simulink model "sampleModel15"  (Simulink 9.1)
settings: Solver=VariableStepAuto  StartTime=0.0  StopTime=10.0  RelTol=1e-3
undefined symbols (not defined in the file): DiscIntNeverNeededParam, magnitude, Newton, Raphson
libraries: simulink x26
settings Model: SuppressorTable="22 serialization::archive 11 0 6 0 0 1 8 0 0 0 0 6 0 0 1 0 21 sampleModel15/cfblk25 0 6 0 0 2 8 0 0 0 0 6 41 Simulink:DataType:WarningOverFlowDetected 0 0 0 6 0  0  0 0 0 0 8 20160608 0 0 0 15 23 17 0 1 40 SimulinkFixedPoint:util:Overflowoccurred 0 0 0  0  8 20160608 0 15 23 17 0 1"  Creator=DELL  LastModifiedBy=DELL
settings DataIOCC: SaveFormat=Dataset
settings OptimizationCC: LifeSpan=auto
settings DebuggingCC: UnderspecifiedInitializationDetection=Simplified  MergeDetectMultiDrivingBlocksExec=error  SFUnexpectedBacktrackingDiag=error  SFNoUnconditionalDefaultTransitionDiag=error  SFExecutionAtInitializationDiag=warning
settings HardwareCC: ProdBitPerPointer=64  ProdBitPerSizeT=64  ProdBitPerPtrDiffT=64  ProdLargestAtomicFloat=Float  ProdIntDivRoundTo=Zero  ProdEndianess=LittleEndian  ProdWordSize=64  ProdHWDeviceType=Intel->x86-64 (Windows64)
settings ModelReferenceCC: PropagateSignalLabelsOutOfModel=on
settings CodeAppCC: StateflowObjectComments=off
settings GRTTargetCC: TargetLangStandard=C99 (ISO)  CombineOutputUpdateFcns=on  GRTInterface=off
settings ConfigComp: CovMetricSettings=dwe  CovHtmlReporting=off  CovSaveCumulativeToWorkspaceVar=off  CovSaveSingleToWorkspaceVar=off  CovExternalEMLEnable=on

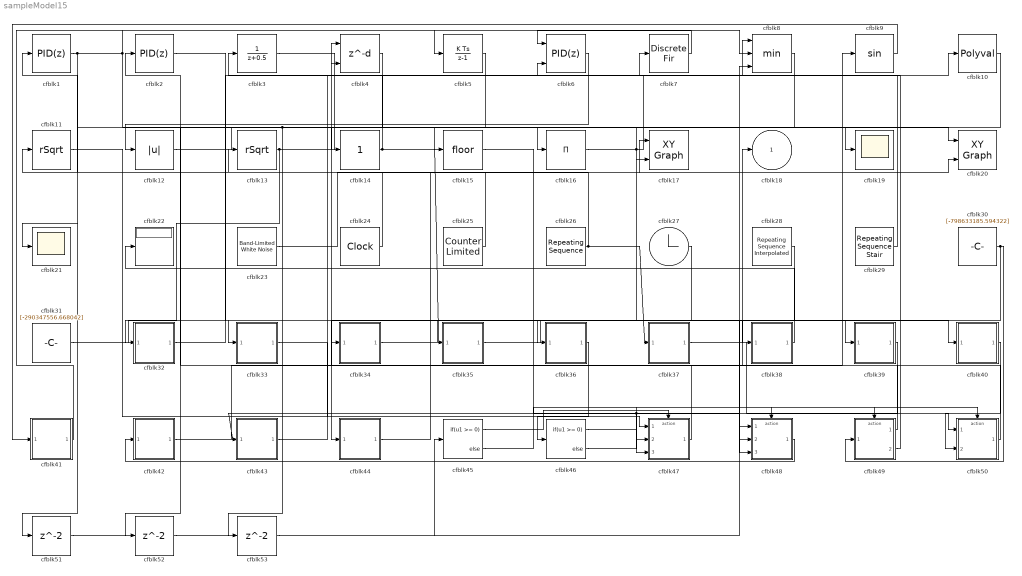
== system sampleModel15 ==
  cfblk1 : simulink/Continuous/PID Controller  Controller=PID  TimeDomain=Discrete-time  SampleTime=1  IntegratorMethod=Forward Euler  FilterMethod=Forward Euler  Form=Parallel  UseFilter=on  ControllerParametersSource=internal  P=1  I=1  D=0  N=100  InitialConditionSource=internal  InitialConditionForIntegrator=0  InitialConditionForFilter=0  ExternalReset=none  LimitOutput=off  UpperSaturationLimit=inf  LowerSaturationLimit=-inf  LinearizeAsGain=off  AntiWindupMode=none  Kb=1  TrackingMode=off  Kt=1  PParamMin=[]  PParamMax=[]  IParamMin=[]  IParamMax=[]  DParamMin=[]  DParamMax=[]  NParamMin=[]  NParamMax=[]  KbParamMin=[]  KbParamMax=[]  KtParamMin=[]  KtParamMax=[]  POutMin=[]  POutMax=[]  IOutMin=[]  IOutMax=[]  DOutMin=[]  DOutMax=[]  NOutMin=[]  NOutMax=[]  KbOutMin=[]  KbOutMax=[]  KtOutMin=[]  KtOutMax=[]  IntegratorOutMin=[]  IntegratorOutMax=[]  FilterOutMin=[]  FilterOutMax=[]  SumOutMin=[]  SumOutMax=[]  SumI1OutMin=[]  SumI1OutMax=[]  SumI2OutMin=[]  SumI2OutMax=[]  SumI3OutMin=[]  SumI3OutMax=[]  SumDOutMin=[]  SumDOutMax=[]  SaturationOutMin=[]  SaturationOutMax=[]  IntegratorContinuousStateAttributes=''  IntegratorStateMustResolveToSignalObject=off  IntegratorRTWStateStorageClass=Auto  FilterContinuousStateAttributes=''  FilterStateMustResolveToSignalObject=off  FilterRTWStateStorageClass=Auto  DifferentiatorICPrevScaledInput=0  DifferentiatorOutMin=[]  DifferentiatorOutMax=[]  FilterDiffOutCoefMin=[]  FilterDiffOutCoefMax=[]  SumDenOutMin=[]  SumDenOutMax=[]  SumNumOutMin=[]  SumNumOutMax=[]  ReciprocalOutMin=[]  ReciprocalOutMax=[]  DivideOutMin=[]  DivideOutMax=[]  TunerSelectOption=Transfer Function Based (PID Tuner App)
  cfblk10 : Polyval  Coefs=[ +2.081618890e-019, -1.441693666e-014, +4.719686976e-010, -8.536869453e-006, +1.621573104e-001, -8.087801117e+001 ]
  cfblk11 : Sqrt  Operator=rSqrt  AlgorithmType=Newton-Raphson  SaturateOnIntegerOverflow=on
  cfblk12 : Abs
  cfblk13 : Sqrt  Operator=rSqrt  AlgorithmType=Newton-Raphson  SaturateOnIntegerOverflow=on
  cfblk14 : simulink/Math Operations/Slider Gain  gain=1  low=0  high=2
  cfblk15 : Rounding
  cfblk16 : Product  Inputs=*
  cfblk17 : simulink/Sinks/XY Graph  xmin=-1  xmax=1  ymin=-1  ymax=1  st=-1
  cfblk19 : Scope
  cfblk2 : simulink/Continuous/PID Controller  Controller=PID  TimeDomain=Discrete-time  SampleTime=1  IntegratorMethod=Forward Euler  FilterMethod=Forward Euler  Form=Parallel  UseFilter=on  ControllerParametersSource=internal  P=1  I=1  D=0  N=100  InitialConditionSource=internal  InitialConditionForIntegrator=0  InitialConditionForFilter=0  ExternalReset=none  LimitOutput=off  UpperSaturationLimit=inf  LowerSaturationLimit=-inf  LinearizeAsGain=off  AntiWindupMode=none  Kb=1  TrackingMode=off  Kt=1  PParamMin=[]  PParamMax=[]  IParamMin=[]  IParamMax=[]  DParamMin=[]  DParamMax=[]  NParamMin=[]  NParamMax=[]  KbParamMin=[]  KbParamMax=[]  KtParamMin=[]  KtParamMax=[]  POutMin=[]  POutMax=[]  IOutMin=[]  IOutMax=[]  DOutMin=[]  DOutMax=[]  NOutMin=[]  NOutMax=[]  KbOutMin=[]  KbOutMax=[]  KtOutMin=[]  KtOutMax=[]  IntegratorOutMin=[]  IntegratorOutMax=[]  FilterOutMin=[]  FilterOutMax=[]  SumOutMin=[]  SumOutMax=[]  SumI1OutMin=[]  SumI1OutMax=[]  SumI2OutMin=[]  SumI2OutMax=[]  SumI3OutMin=[]  SumI3OutMax=[]  SumDOutMin=[]  SumDOutMax=[]  SaturationOutMin=[]  SaturationOutMax=[]  IntegratorContinuousStateAttributes=''  IntegratorStateMustResolveToSignalObject=off  IntegratorRTWStateStorageClass=Auto  FilterContinuousStateAttributes=''  FilterStateMustResolveToSignalObject=off  FilterRTWStateStorageClass=Auto  DifferentiatorICPrevScaledInput=0  DifferentiatorOutMin=[]  DifferentiatorOutMax=[]  FilterDiffOutCoefMin=[]  FilterDiffOutCoefMax=[]  SumDenOutMin=[]  SumDenOutMax=[]  SumNumOutMin=[]  SumNumOutMax=[]  ReciprocalOutMin=[]  ReciprocalOutMax=[]  DivideOutMin=[]  DivideOutMax=[]  TunerSelectOption=Transfer Function Based (PID Tuner App)
  cfblk20 : simulink/Sinks/XY Graph  xmin=-1  xmax=1  ymin=-1  ymax=1  st=-1
  cfblk21 : Scope
  cfblk22 : Display
  cfblk23 : simulink/Sources/Band-Limited White Noise  Cov=[4615233474.301985]  Ts=0.1  seed=[9049221695.000000]
  cfblk24 : DigitalClock
  cfblk25 : simulink/Sources/Counter Limited  uplimit=[387.000000]  tsamp=-1
  cfblk26 : simulink/Sources/Repeating Sequence  rep_seq_t=[0 2]  rep_seq_y=[206033104.560979, 120638017.420712]
  cfblk27 : Clock
  cfblk28 : simulink/Sources/Repeating Sequence Interpolated  OutValues=[691679511.220975, -430390090.474105, 326636995.361738, 204516353.053731, 312925893.425582]  TimeValues=[0 0.1 0.5 0.6 1].'  LookUpMeth=Use Input Nearest  tsamp=0.01  OutMin=[]  OutMax=[]  OutDataTypeStr=double  OutputDataTypeScalingMode=double  OutDataType=fixdt(0,8)  OutScaling=2^-10
  cfblk29 : simulink/Sources/Repeating Sequence Stair  OutValues=[-336712385.924395, -623605342.299720]  tsamp=-1  OutMin=[]  OutMax=[]  OutDataTypeStr=double  OutputDataTypeScalingMode=double  OutDataType=fixdt(0,8)  ConRadixGroup=Best Precision: Vector-wise  OutScaling=2^-12
  cfblk3 : DiscreteTransferFcn  SampleTime=1
  cfblk30 : Constant  Value=[-798633185.594322]  SampleTime=1
  cfblk31 : Constant  Value=[-290347556.668042]  SampleTime=1
  cfblk32 : Subsystem
  cfblk33 : Subsystem
  cfblk34 : Subsystem
  cfblk35 : Subsystem
  cfblk36 : Subsystem
  cfblk37 : Subsystem
  cfblk38 : Subsystem
  cfblk39 : Subsystem
  cfblk4 : Delay  DelayLengthSource=Input port  SampleTime=1
      settings: InputPortMap=u0,p1
  cfblk40 : Subsystem
  cfblk41 : Subsystem
  cfblk42 : Subsystem
  cfblk43 : Subsystem
  cfblk44 : Subsystem
  cfblk45 : If  IfExpression=u1 >= 0  SampleTime=1
  cfblk46 : If  IfExpression=u1 >= 0  SampleTime=1
  cfblk47 : Subsystem  TreatAsAtomicUnit=on
  cfblk48 : Subsystem  TreatAsAtomicUnit=on
  cfblk49 : Subsystem  TreatAsAtomicUnit=on
  cfblk5 : DiscreteIntegrator  ICPrevOutput=DiscIntNeverNeededParam  ICPrevScaledInput=DiscIntNeverNeededParam
  cfblk50 : Subsystem  TreatAsAtomicUnit=on
  cfblk51 : Delay  SampleTime=1
  cfblk52 : Delay  SampleTime=1
  cfblk53 : Delay  SampleTime=1
  cfblk6 : simulink/Continuous/PID Controller (2DOF)  Controller=PID  TimeDomain=Discrete-time  SampleTime=1  IntegratorMethod=Forward Euler  FilterMethod=Forward Euler  Form=Parallel  UseFilter=on  ControllerParametersSource=internal  P=1  I=1  D=0  N=100  b=1  c=1  InitialConditionSource=internal  InitialConditionForIntegrator=0  InitialConditionForFilter=0  ExternalReset=none  LimitOutput=off  UpperSaturationLimit=inf  LowerSaturationLimit=-inf  LinearizeAsGain=off  AntiWindupMode=none  Kb=1  TrackingMode=off  Kt=1  PParamMin=[]  PParamMax=[]  IParamMin=[]  IParamMax=[]  DParamMin=[]  DParamMax=[]  NParamMin=[]  NParamMax=[]  bParamMin=[]  bParamMax=[]  cParamMin=[]  cParamMax=[]  KbParamMin=[]  KbParamMax=[]  KtParamMin=[]  KtParamMax=[]  POutMin=[]  POutMax=[]  IOutMin=[]  IOutMax=[]  DOutMin=[]  DOutMax=[]  NOutMin=[]  NOutMax=[]  bOutMin=[]  bOutMax=[]  cOutMin=[]  cOutMax=[]  KbOutMin=[]  KbOutMax=[]  KtOutMin=[]  KtOutMax=[]  IntegratorOutMin=[]  IntegratorOutMax=[]  FilterOutMin=[]  FilterOutMax=[]  SumOutMin=[]  SumOutMax=[]  Sum1OutMin=[]  Sum1OutMax=[]  Sum2OutMin=[]  Sum2OutMax=[]  Sum3OutMin=[]  Sum3OutMax=[]  SumI1OutMin=[]  SumI1OutMax=[]  SumI2OutMin=[]  SumI2OutMax=[]  SumI3OutMin=[]  SumI3OutMax=[]  SumDOutMin=[]  SumDOutMax=[]  SaturationOutMin=[]  SaturationOutMax=[]  IntegratorContinuousStateAttributes=''  IntegratorStateMustResolveToSignalObject=off  IntegratorRTWStateStorageClass=Auto  FilterContinuousStateAttributes=''  FilterStateMustResolveToSignalObject=off  FilterRTWStateStorageClass=Auto  DifferentiatorICPrevScaledInput=0  DifferentiatorOutMin=[]  DifferentiatorOutMax=[]  FilterDiffOutCoefMin=[]  FilterDiffOutCoefMax=[]  SumDenOutMin=[]  SumDenOutMax=[]  SumNumOutMin=[]  SumNumOutMax=[]  ReciprocalOutMin=[]  ReciprocalOutMax=[]  DivideOutMin=[]  DivideOutMax=[]  TunerSelectOption=Transfer Function Based (PID Tuner App)
  cfblk7 : DiscreteFir  SampleTime=1
  cfblk8 : MinMax  Inputs=3
  cfblk9 : Trigonometry
  cfblk18 : Outport
  wires:
  cfblk25/1 -> cfblk11/1
  cfblk48/1(cfblk2) -> cfblk42/1(cfblk1)
  cfblk13/1 -> cfblk20/1, cfblk32/1(cfblk1)
  cfblk12/1 -> cfblk19/1
  cfblk6/1 -> cfblk12/1
  cfblk29/1 -> cfblk7/1
  cfblk47/1(cfblk2) -> cfblk4/1
  cfblk7/1 -> cfblk6/1
  cfblk35/1(cfblk2) -> cfblk39/1(cfblk1)
  cfblk3/1 -> cfblk16/1
  cfblk24/1 -> cfblk1/1
  cfblk27/1 -> cfblk44/1(cfblk1)
  cfblk41/1(cfblk2) -> cfblk5/1
  cfblk26/1 -> cfblk37/1(cfblk1), cfblk13/1
  cfblk31/1 -> cfblk33/1(cfblk1)
  cfblk34/1(cfblk2) -> cfblk36/1(cfblk1)
  cfblk42/1(cfblk2) -> cfblk9/1
  cfblk16/1 -> cfblk10/1, cfblk40/1(cfblk1)
  cfblk10/1 -> cfblk14/1
  cfblk49/1(cfblk2) -> cfblk2/1
  cfblk28/1 -> cfblk34/1(cfblk1)
  cfblk14/1 -> cfblk35/1(cfblk1), cfblk4/2
  cfblk50/1(cfblk2) -> cfblk18/1
  cfblk38/1(cfblk2) -> cfblk22/1
  cfblk39/1(cfblk2) -> cfblk43/1(cfblk1), cfblk47/3(cfblk11)
  cfblk8/1 -> cfblk15/1
  cfblk5/1 -> cfblk52/1, cfblk53/1
  cfblk37/1(cfblk2) -> cfblk50/1(cfblk1)
  cfblk43/1(cfblk2) -> cfblk6/2
  cfblk30/1 -> cfblk49/1(cfblk1), cfblk48/3(cfblk7)
  cfblk23/1 -> cfblk20/2
  cfblk9/1 -> cfblk41/1(cfblk1)
  cfblk49/2(cfblk15) -> cfblk3/1
  cfblk40/1(cfblk2) -> cfblk50/2(cfblk12)
  cfblk15/1 -> cfblk48/2(cfblk6)
  cfblk32/1(cfblk2) -> cfblk8/1
  cfblk36/1(cfblk2) -> cfblk46/1
  cfblk33/1(cfblk2) -> cfblk47/1(cfblk1)
  cfblk2/1 -> cfblk38/1(cfblk1)
  cfblk44/1(cfblk2) -> cfblk17/1
  cfblk1/1 -> cfblk17/2, cfblk8/2, cfblk21/1
  cfblk11/1 -> cfblk47/2(cfblk10)
  cfblk45/1 -> cfblk47/Action
  cfblk45/2 -> cfblk48/Action
  cfblk46/1 -> cfblk49/Action
  cfblk46/2 -> cfblk50/Action
  cfblk4/1 -> cfblk51/1
  cfblk51/1 -> cfblk48/1(cfblk1)
  cfblk52/1 -> cfblk45/1
  cfblk53/1 -> cfblk8/3

== system sampleModel15/cfblk32 ==
  cfblk1 : Inport
  cfblk2 : Outport
  wires:
  cfblk1/1 -> cfblk2/1

== system sampleModel15/cfblk33 ==
  cfblk1 : Inport
  cfblk2 : Outport
  wires:
  cfblk1/1 -> cfblk2/1

== system sampleModel15/cfblk34 ==
  cfblk1 : Inport
  cfblk2 : Outport
  wires:
  cfblk1/1 -> cfblk2/1

== system sampleModel15/cfblk35 ==
  cfblk1 : Inport
  cfblk2 : Outport
  wires:
  cfblk1/1 -> cfblk2/1

== system sampleModel15/cfblk36 ==
  cfblk1 : Inport
  cfblk2 : Outport
  wires:
  cfblk1/1 -> cfblk2/1

== system sampleModel15/cfblk37 ==
  cfblk1 : Inport
  cfblk2 : Outport
  wires:
  cfblk1/1 -> cfblk2/1

== system sampleModel15/cfblk38 ==
  cfblk1 : Inport
  cfblk2 : Outport
  wires:
  cfblk1/1 -> cfblk2/1

== system sampleModel15/cfblk39 ==
  cfblk1 : Inport
  cfblk2 : Outport
  wires:
  cfblk1/1 -> cfblk2/1

== system sampleModel15/cfblk40 ==
  cfblk1 : Inport
  cfblk2 : Outport
  wires:
  cfblk1/1 -> cfblk2/1

== system sampleModel15/cfblk41 ==
  cfblk1 : Inport
  cfblk2 : Outport
  wires:
  cfblk1/1 -> cfblk2/1

== system sampleModel15/cfblk42 ==
  cfblk1 : Inport
  cfblk2 : Outport
  wires:
  cfblk1/1 -> cfblk2/1

== system sampleModel15/cfblk43 ==
  cfblk1 : Inport
  cfblk2 : Outport
  wires:
  cfblk1/1 -> cfblk2/1

== system sampleModel15/cfblk44 ==
  cfblk1 : Inport
  cfblk2 : Outport
  wires:
  cfblk1/1 -> cfblk2/1

== system sampleModel15/cfblk47 ==
  cfblk1 : Inport
  cfblk10 : Inport  Port=2
  cfblk11 : Inport  Port=3
  Action Port : ActionPort  ActionType=then
  cfblk12 : Delay
  cfblk3 : Delay
  cfblk4 : DiscreteZeroPole  Poles=[0 0.5]  Gain=1  SampleTime=-1
  cfblk5 : simulink/Continuous/PID Controller  Controller=PID  TimeDomain=Discrete-time  SampleTime=-1  IntegratorMethod=Forward Euler  FilterMethod=Forward Euler  Form=Parallel  UseFilter=on  ControllerParametersSource=internal  P=1  I=1  D=0  N=100  InitialConditionSource=internal  InitialConditionForIntegrator=0  InitialConditionForFilter=0  ExternalReset=none  LimitOutput=off  UpperSaturationLimit=inf  LowerSaturationLimit=-inf  LinearizeAsGain=off  AntiWindupMode=none  Kb=1  TrackingMode=off  Kt=1  PParamMin=[]  PParamMax=[]  IParamMin=[]  IParamMax=[]  DParamMin=[]  DParamMax=[]  NParamMin=[]  NParamMax=[]  KbParamMin=[]  KbParamMax=[]  KtParamMin=[]  KtParamMax=[]  POutMin=[]  POutMax=[]  IOutMin=[]  IOutMax=[]  DOutMin=[]  DOutMax=[]  NOutMin=[]  NOutMax=[]  KbOutMin=[]  KbOutMax=[]  KtOutMin=[]  KtOutMax=[]  IntegratorOutMin=[]  IntegratorOutMax=[]  FilterOutMin=[]  FilterOutMax=[]  SumOutMin=[]  SumOutMax=[]  SumI1OutMin=[]  SumI1OutMax=[]  SumI2OutMin=[]  SumI2OutMax=[]  SumI3OutMin=[]  SumI3OutMax=[]  SumDOutMin=[]  SumDOutMax=[]  SaturationOutMin=[]  SaturationOutMax=[]  IntegratorContinuousStateAttributes=''  IntegratorStateMustResolveToSignalObject=off  IntegratorRTWStateStorageClass=Auto  FilterContinuousStateAttributes=''  FilterStateMustResolveToSignalObject=off  FilterRTWStateStorageClass=Auto  DifferentiatorICPrevScaledInput=0  DifferentiatorOutMin=[]  DifferentiatorOutMax=[]  FilterDiffOutCoefMin=[]  FilterDiffOutCoefMax=[]  SumDenOutMin=[]  SumDenOutMax=[]  SumNumOutMin=[]  SumNumOutMax=[]  ReciprocalOutMin=[]  ReciprocalOutMax=[]  DivideOutMin=[]  DivideOutMax=[]  TunerSelectOption=Transfer Function Based (PID Tuner App)
  cfblk6 : ComplexToMagnitudeAngle
  cfblk7 : Constant  Value=[-442457058.559597]  SampleTime=1
  cfblk8 : Constant  Value=[-425591701.658393]  SampleTime=1
  cfblk9 : Subsystem
  cfblk2 : Outport
  wires:
  cfblk5/1 -> cfblk9/1(cfblk1)
  cfblk4/1 -> cfblk5/1
  cfblk9/1(cfblk2) -> cfblk6/1
  cfblk1/1 -> cfblk2/1
  cfblk6/2 -> cfblk3/1
  cfblk6/1 -> cfblk12/1
  cfblk12/1 -> cfblk4/1

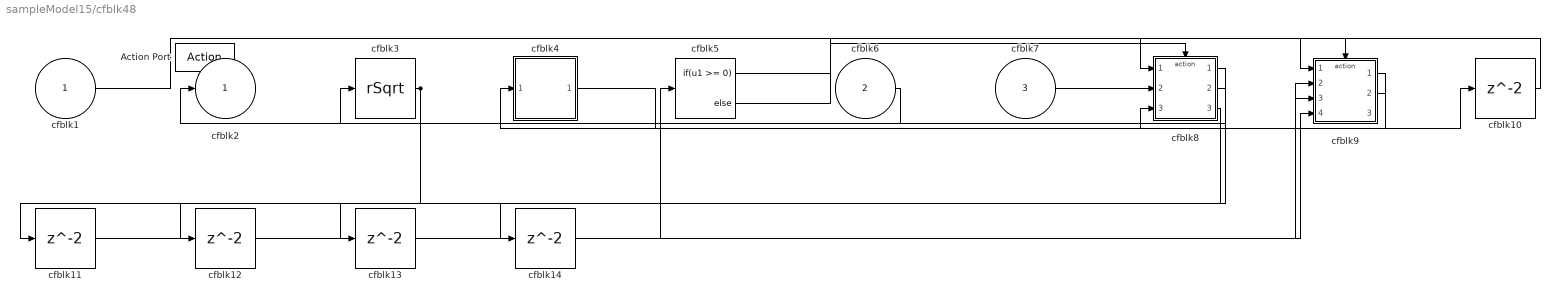
== system sampleModel15/cfblk48 ==
  cfblk1 : Inport
  cfblk6 : Inport  Port=2
  cfblk7 : Inport  Port=3
  Action Port : ActionPort  ActionType=else
  cfblk{10..14} (5 alike) : Delay
  cfblk3 : Sqrt  Operator=rSqrt  AlgorithmType=Newton-Raphson  SaturateOnIntegerOverflow=on
  cfblk4 : Subsystem
  cfblk5 : If  IfExpression=u1 >= 0  SampleTime=1
  cfblk8 : Subsystem  TreatAsAtomicUnit=on
  cfblk9 : Subsystem  TreatAsAtomicUnit=on
  cfblk2 : Outport
  wires:
  cfblk7/1 -> cfblk8/2(cfblk12)
  cfblk1/1 -> cfblk9/1(cfblk1)
  cfblk3/1 -> cfblk12/1, cfblk13/1
  cfblk9/1(cfblk2) -> cfblk4/1(cfblk1)
  cfblk6/1 -> cfblk2/1
  cfblk9/2(cfblk15) -> cfblk8/3(cfblk13)
  cfblk8/2(cfblk14) -> cfblk3/1
  cfblk5/1 -> cfblk8/Action
  cfblk5/2 -> cfblk9/Action
  cfblk4/1(cfblk2) -> cfblk10/1
  cfblk10/1 -> cfblk8/1(cfblk1)
  cfblk8/1(cfblk2) -> cfblk11/1
  cfblk11/1 -> cfblk9/2(cfblk12)
  cfblk12/1 -> cfblk5/1
  cfblk13/1 -> cfblk9/4(cfblk14)
  cfblk8/3(cfblk15) -> cfblk14/1
  cfblk14/1 -> cfblk9/3(cfblk13)

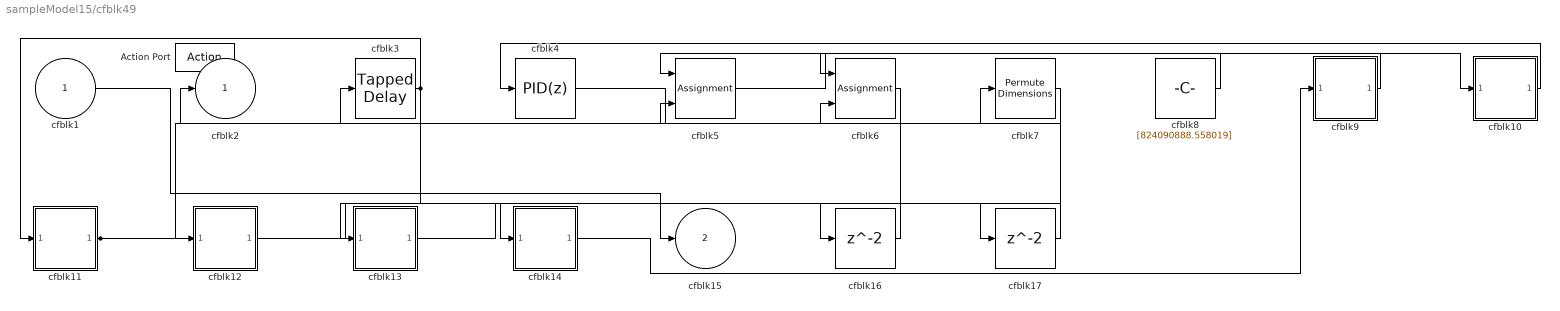
== system sampleModel15/cfblk49 ==
  cfblk1 : Inport
  Action Port : ActionPort  ActionType=then
  cfblk10 : Subsystem
  cfblk11 : Subsystem
  cfblk12 : Subsystem
  cfblk13 : Subsystem
  cfblk14 : Subsystem
  cfblk16 : Delay
  cfblk17 : Delay
  cfblk3 : simulink/Discrete/Tapped Delay  vinit=0.0  samptime=-1  NumDelays=1  DelayOrder=Oldest  includeCurrent=off
  cfblk4 : simulink/Continuous/PID Controller  Controller=PID  TimeDomain=Discrete-time  SampleTime=-1  IntegratorMethod=Forward Euler  FilterMethod=Forward Euler  Form=Parallel  UseFilter=on  ControllerParametersSource=internal  P=1  I=1  D=0  N=100  InitialConditionSource=internal  InitialConditionForIntegrator=0  InitialConditionForFilter=0  ExternalReset=none  LimitOutput=off  UpperSaturationLimit=inf  LowerSaturationLimit=-inf  LinearizeAsGain=off  AntiWindupMode=none  Kb=1  TrackingMode=off  Kt=1  PParamMin=[]  PParamMax=[]  IParamMin=[]  IParamMax=[]  DParamMin=[]  DParamMax=[]  NParamMin=[]  NParamMax=[]  KbParamMin=[]  KbParamMax=[]  KtParamMin=[]  KtParamMax=[]  POutMin=[]  POutMax=[]  IOutMin=[]  IOutMax=[]  DOutMin=[]  DOutMax=[]  NOutMin=[]  NOutMax=[]  KbOutMin=[]  KbOutMax=[]  KtOutMin=[]  KtOutMax=[]  IntegratorOutMin=[]  IntegratorOutMax=[]  FilterOutMin=[]  FilterOutMax=[]  SumOutMin=[]  SumOutMax=[]  SumI1OutMin=[]  SumI1OutMax=[]  SumI2OutMin=[]  SumI2OutMax=[]  SumI3OutMin=[]  SumI3OutMax=[]  SumDOutMin=[]  SumDOutMax=[]  SaturationOutMin=[]  SaturationOutMax=[]  IntegratorContinuousStateAttributes=''  IntegratorStateMustResolveToSignalObject=off  IntegratorRTWStateStorageClass=Auto  FilterContinuousStateAttributes=''  FilterStateMustResolveToSignalObject=off  FilterRTWStateStorageClass=Auto  DifferentiatorICPrevScaledInput=0  DifferentiatorOutMin=[]  DifferentiatorOutMax=[]  FilterDiffOutCoefMin=[]  FilterDiffOutCoefMax=[]  SumDenOutMin=[]  SumDenOutMax=[]  SumNumOutMin=[]  SumNumOutMax=[]  ReciprocalOutMin=[]  ReciprocalOutMax=[]  DivideOutMin=[]  DivideOutMax=[]  TunerSelectOption=Transfer Function Based (PID Tuner App)
  cfblk5 : Assignment  DiagnosticForDimensions=Warning  IndexOptions=Index vector (dialog)  Indices=1  OutputSizes=1
  cfblk6 : Assignment  DiagnosticForDimensions=Warning  IndexOptions=Index vector (dialog)  Indices=1  OutputSizes=1
  cfblk7 : PermuteDimensions
  cfblk8 : Constant  Value=[824090888.558019]  SampleTime=1
  cfblk9 : Subsystem
  cfblk2 : Outport
  cfblk15 : Outport  Port=2
  wires:
  cfblk11/1(cfblk2) -> cfblk12/1(cfblk1), cfblk6/2
  cfblk6/1 -> cfblk2/1
  cfblk3/1 -> cfblk11/1(cfblk1), cfblk13/1(cfblk1)
  cfblk5/1 -> cfblk10/1(cfblk1)
  cfblk12/1(cfblk2) -> cfblk14/1(cfblk1)
  cfblk8/1 -> cfblk6/1
  cfblk1/1 -> cfblk15/1
  cfblk9/1(cfblk2) -> cfblk5/1
  cfblk4/1 -> cfblk7/1
  cfblk10/1(cfblk2) -> cfblk4/1
  cfblk14/1(cfblk2) -> cfblk9/1(cfblk1)
  cfblk7/1 -> cfblk16/1
  cfblk16/1 -> cfblk5/2
  cfblk13/1(cfblk2) -> cfblk17/1
  cfblk17/1 -> cfblk3/1

== system sampleModel15/cfblk50 ==
  cfblk1 : Inport
  cfblk12 : Inport  Port=2
  Action Port : ActionPort  ActionType=else
  cfblk10 : Subsystem
  cfblk11 : Subsystem
  cfblk13 : Delay
  cfblk3 : UnitDelay  SampleTime=-1
  cfblk4 : Sum  Inputs=-+
  cfblk5 : ComplexToMagnitudeAngle
  cfblk6 : simulink/Math Operations/MinMax Running Resettable  Function=min  vinit=0.0
  cfblk7 : Assignment  DiagnosticForDimensions=Warning  IndexOptions=Index vector (dialog)  Indices=1  OutputSizes=1
  cfblk8 : Constant  Value=[310628600.138073]  SampleTime=1
  cfblk9 : Constant  Value=[-993756271.282597]  SampleTime=1
  cfblk2 : Outport
  wires:
  cfblk10/1(cfblk2) -> cfblk2/1
  cfblk11/1(cfblk2) -> cfblk4/1
  cfblk6/1 -> cfblk7/1
  cfblk1/1 -> cfblk5/1
  cfblk8/1 -> cfblk11/1(cfblk1)
  cfblk3/1 -> cfblk4/2
  cfblk12/1 -> cfblk3/1
  cfblk5/1 -> cfblk6/1
  cfblk4/1 -> cfblk10/1(cfblk1)
  cfblk9/1 -> cfblk7/2
  cfblk7/1 -> cfblk13/1
  cfblk13/1 -> cfblk6/2

== system sampleModel15/cfblk47/cfblk9 ==
  cfblk1 : Inport
  cfblk2 : Outport
  wires:
  cfblk1/1 -> cfblk2/1

== system sampleModel15/cfblk48/cfblk4 ==
  cfblk1 : Inport
  cfblk2 : Outport
  wires:
  cfblk1/1 -> cfblk2/1

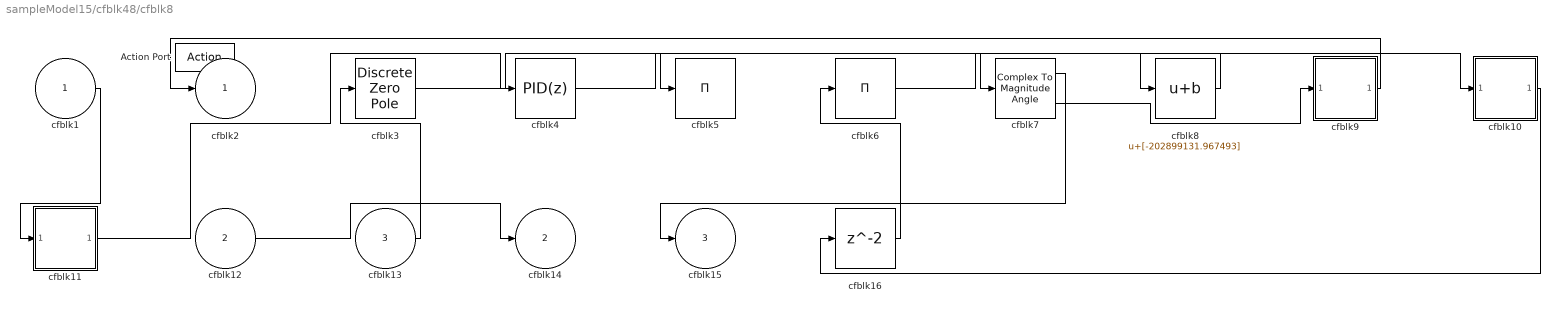
== system sampleModel15/cfblk48/cfblk8 ==
  cfblk1 : Inport
  cfblk12 : Inport  Port=2
  cfblk13 : Inport  Port=3
  Action Port : ActionPort  ActionType=then
  cfblk10 : Subsystem
  cfblk11 : Subsystem
  cfblk16 : Delay
  cfblk3 : DiscreteZeroPole  Poles=[0 0.5]  Gain=1  SampleTime=-1
  cfblk4 : simulink/Continuous/PID Controller  Controller=PID  TimeDomain=Discrete-time  SampleTime=-1  IntegratorMethod=Forward Euler  FilterMethod=Forward Euler  Form=Parallel  UseFilter=on  ControllerParametersSource=internal  P=1  I=1  D=0  N=100  InitialConditionSource=internal  InitialConditionForIntegrator=0  InitialConditionForFilter=0  ExternalReset=none  LimitOutput=off  UpperSaturationLimit=inf  LowerSaturationLimit=-inf  LinearizeAsGain=off  AntiWindupMode=none  Kb=1  TrackingMode=off  Kt=1  PParamMin=[]  PParamMax=[]  IParamMin=[]  IParamMax=[]  DParamMin=[]  DParamMax=[]  NParamMin=[]  NParamMax=[]  KbParamMin=[]  KbParamMax=[]  KtParamMin=[]  KtParamMax=[]  POutMin=[]  POutMax=[]  IOutMin=[]  IOutMax=[]  DOutMin=[]  DOutMax=[]  NOutMin=[]  NOutMax=[]  KbOutMin=[]  KbOutMax=[]  KtOutMin=[]  KtOutMax=[]  IntegratorOutMin=[]  IntegratorOutMax=[]  FilterOutMin=[]  FilterOutMax=[]  SumOutMin=[]  SumOutMax=[]  SumI1OutMin=[]  SumI1OutMax=[]  SumI2OutMin=[]  SumI2OutMax=[]  SumI3OutMin=[]  SumI3OutMax=[]  SumDOutMin=[]  SumDOutMax=[]  SaturationOutMin=[]  SaturationOutMax=[]  IntegratorContinuousStateAttributes=''  IntegratorStateMustResolveToSignalObject=off  IntegratorRTWStateStorageClass=Auto  FilterContinuousStateAttributes=''  FilterStateMustResolveToSignalObject=off  FilterRTWStateStorageClass=Auto  DifferentiatorICPrevScaledInput=0  DifferentiatorOutMin=[]  DifferentiatorOutMax=[]  FilterDiffOutCoefMin=[]  FilterDiffOutCoefMax=[]  SumDenOutMin=[]  SumDenOutMax=[]  SumNumOutMin=[]  SumNumOutMax=[]  ReciprocalOutMin=[]  ReciprocalOutMax=[]  DivideOutMin=[]  DivideOutMax=[]  TunerSelectOption=Transfer Function Based (PID Tuner App)
  cfblk5 : Product  Inputs=*
  cfblk6 : Product  Inputs=*
  cfblk7 : ComplexToMagnitudeAngle
  cfblk8 : Bias  Bias=[-202899131.967493]
  cfblk9 : Subsystem
  cfblk2 : Outport
  cfblk14 : Outport  Port=2
  cfblk15 : Outport  Port=3
  wires:
  cfblk12/1 -> cfblk14/1
  cfblk8/1 -> cfblk7/1
  cfblk7/1 -> cfblk15/1
  cfblk7/2 -> cfblk9/1(cfblk1)
  cfblk3/1 -> cfblk5/1
  cfblk4/1 -> cfblk8/1
  cfblk13/1 -> cfblk3/1
  cfblk9/1(cfblk2) -> cfblk2/1
  cfblk1/1 -> cfblk11/1(cfblk1)
  cfblk11/1(cfblk2) -> cfblk4/1
  cfblk6/1 -> cfblk10/1(cfblk1)
  cfblk10/1(cfblk2) -> cfblk16/1
  cfblk16/1 -> cfblk6/1

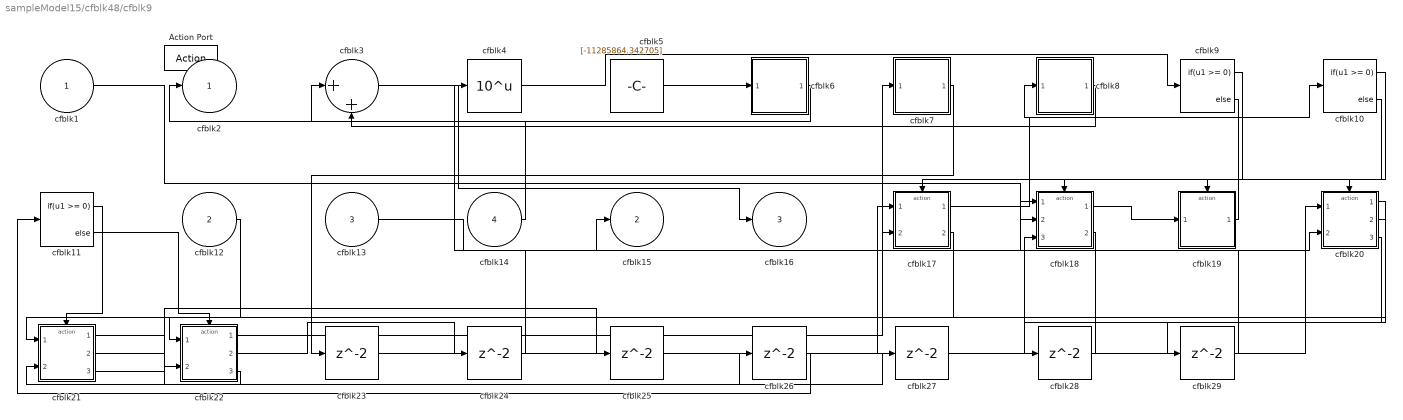
== system sampleModel15/cfblk48/cfblk9 ==
  cfblk1 : Inport
  cfblk12 : Inport  Port=2
  cfblk13 : Inport  Port=3
  cfblk14 : Inport  Port=4
  Action Port : ActionPort  ActionType=else
  cfblk10 : If  IfExpression=u1 >= 0  SampleTime=1
  cfblk11 : If  IfExpression=u1 >= 0  SampleTime=1
  cfblk17 : Subsystem  TreatAsAtomicUnit=on
  cfblk18 : Subsystem  TreatAsAtomicUnit=on
  cfblk19 : Subsystem  TreatAsAtomicUnit=on
  cfblk20 : Subsystem  TreatAsAtomicUnit=on
  cfblk21 : Subsystem  TreatAsAtomicUnit=on
  cfblk22 : Subsystem  TreatAsAtomicUnit=on
  cfblk{23..29} (7 alike) : Delay
  cfblk3 : Sum  Inputs=|++
  cfblk4 : Math  Operator=10^u  SaturateOnIntegerOverflow=on
  cfblk5 : Constant  Value=[-11285864.342705]  SampleTime=1
  cfblk6 : Subsystem
  cfblk7 : Subsystem
  cfblk8 : Subsystem
  cfblk9 : If  IfExpression=u1 >= 0  SampleTime=1
  cfblk2 : Outport
  cfblk15 : Outport  Port=2
  cfblk16 : Outport  Port=3
  wires:
  cfblk5/1 -> cfblk6/1(cfblk1)
  cfblk22/1(cfblk2) -> cfblk7/1(cfblk1)
  cfblk17/1(cfblk2) -> cfblk10/1
  cfblk6/1(cfblk2) -> cfblk2/1
  cfblk12/1 -> cfblk21/1(cfblk1)
  cfblk14/1 -> cfblk3/1
  cfblk4/1 -> cfblk9/1
  cfblk13/1 -> cfblk20/2(cfblk11)
  cfblk3/1 -> cfblk16/1
  cfblk17/2(cfblk15) -> cfblk22/1(cfblk1)
  cfblk22/3(cfblk15) -> cfblk21/2(cfblk14)
  cfblk20/1(cfblk2) -> cfblk22/2(cfblk13)
  cfblk19/1(cfblk2) -> cfblk8/1(cfblk1)
  cfblk8/1(cfblk2) -> cfblk3/2
  cfblk18/1(cfblk2) -> cfblk19/1(cfblk1)
  cfblk1/1 -> cfblk18/2(cfblk14)
  cfblk18/2(cfblk16) -> cfblk15/1
  cfblk9/1 -> cfblk17/Action
  cfblk9/2 -> cfblk18/Action
  cfblk10/1 -> cfblk19/Action
  cfblk10/2 -> cfblk20/Action
  cfblk11/1 -> cfblk21/Action
  cfblk11/2 -> cfblk22/Action
  cfblk7/1(cfblk2) -> cfblk23/1
  cfblk23/1 -> cfblk17/1(cfblk1)
  cfblk22/2(cfblk14) -> cfblk24/1
  cfblk24/1 -> cfblk4/1
  cfblk21/1(cfblk2) -> cfblk25/1
  cfblk25/1 -> cfblk20/1(cfblk1)
  cfblk21/2(cfblk15) -> cfblk26/1
  cfblk26/1 -> cfblk11/1
  cfblk21/3(cfblk16) -> cfblk27/1
  cfblk27/1 -> cfblk18/3(cfblk15)
  cfblk20/2(cfblk12) -> cfblk28/1
  cfblk28/1 -> cfblk17/2(cfblk14)
  cfblk20/3(cfblk13) -> cfblk29/1
  cfblk29/1 -> cfblk18/1(cfblk1)

== system sampleModel15/cfblk49/cfblk10 ==
  cfblk1 : Inport
  cfblk2 : Outport
  wires:
  cfblk1/1 -> cfblk2/1

== system sampleModel15/cfblk49/cfblk11 ==
  cfblk1 : Inport
  cfblk2 : Outport
  wires:
  cfblk1/1 -> cfblk2/1

== system sampleModel15/cfblk49/cfblk12 ==
  cfblk1 : Inport
  cfblk2 : Outport
  wires:
  cfblk1/1 -> cfblk2/1

== system sampleModel15/cfblk49/cfblk13 ==
  cfblk1 : Inport
  cfblk2 : Outport
  wires:
  cfblk1/1 -> cfblk2/1

== system sampleModel15/cfblk49/cfblk14 ==
  cfblk1 : Inport
  cfblk2 : Outport
  wires:
  cfblk1/1 -> cfblk2/1

== system sampleModel15/cfblk49/cfblk9 ==
  cfblk1 : Inport
  cfblk2 : Outport
  wires:
  cfblk1/1 -> cfblk2/1

== system sampleModel15/cfblk50/cfblk10 ==
  cfblk1 : Inport
  cfblk2 : Outport
  wires:
  cfblk1/1 -> cfblk2/1

== system sampleModel15/cfblk50/cfblk11 ==
  cfblk1 : Inport
  cfblk2 : Outport
  wires:
  cfblk1/1 -> cfblk2/1

== system sampleModel15/cfblk48/cfblk8/cfblk10 ==
  cfblk1 : Inport
  cfblk2 : Outport
  wires:
  cfblk1/1 -> cfblk2/1

== system sampleModel15/cfblk48/cfblk8/cfblk11 ==
  cfblk1 : Inport
  cfblk2 : Outport
  wires:
  cfblk1/1 -> cfblk2/1

== system sampleModel15/cfblk48/cfblk8/cfblk9 ==
  cfblk1 : Inport
  cfblk2 : Outport
  wires:
  cfblk1/1 -> cfblk2/1

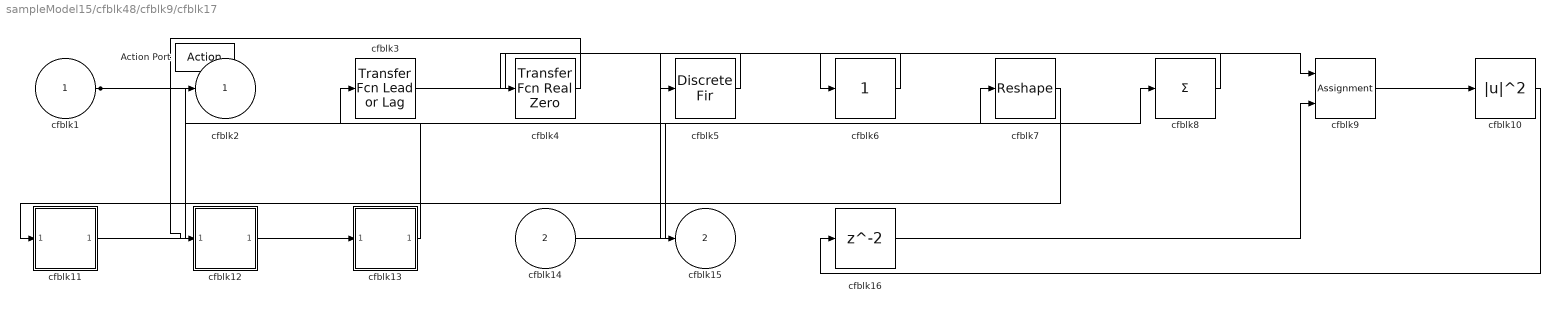
== system sampleModel15/cfblk48/cfblk9/cfblk17 ==
  cfblk1 : Inport
  cfblk14 : Inport  Port=2
  Action Port : ActionPort  ActionType=then
  cfblk10 : Math  Operator=magnitude^2  SaturateOnIntegerOverflow=on
  cfblk11 : Subsystem
  cfblk12 : Subsystem
  cfblk13 : Subsystem
  cfblk16 : Delay
  cfblk3 : simulink/Discrete/Transfer Fcn Lead or Lag  PoleZ=0.95  ZeroZ=0.75  ICPrevOutput=0.0  ICPrevInput=0.0  DoSatur=off
      settings: SourceProductName=Simulink  SourceProductBaseCode=SL
  cfblk4 : simulink/Discrete/Transfer Fcn Real Zero  ZeroZ=0.75  ICPrevInput=0.0  DoSatur=off
      settings: SourceProductName=Simulink  SourceProductBaseCode=SL
  cfblk5 : DiscreteFir
  cfblk6 : simulink/Math Operations/Slider Gain  gain=1  low=0  high=2
  cfblk7 : Reshape
  cfblk8 : Sum  Inputs=+
  cfblk9 : Assignment  DiagnosticForDimensions=Warning  IndexOptions=Index vector (dialog)  Indices=1  OutputSizes=1
  cfblk2 : Outport
  cfblk15 : Outport  Port=2
  wires:
  cfblk14/1 -> cfblk8/1
  cfblk12/1(cfblk2) -> cfblk13/1(cfblk1)
  cfblk6/1 -> cfblk15/1
  cfblk11/1(cfblk2) -> cfblk5/1
  cfblk13/1(cfblk2) -> cfblk3/1
  cfblk4/1 -> cfblk12/1(cfblk1)
  cfblk8/1 -> cfblk6/1
  cfblk9/1 -> cfblk10/1
  cfblk1/1 -> cfblk7/1, cfblk2/1
  cfblk3/1 -> cfblk9/1
  cfblk7/1 -> cfblk11/1(cfblk1)
  cfblk5/1 -> cfblk4/1
  cfblk10/1 -> cfblk16/1
  cfblk16/1 -> cfblk9/2

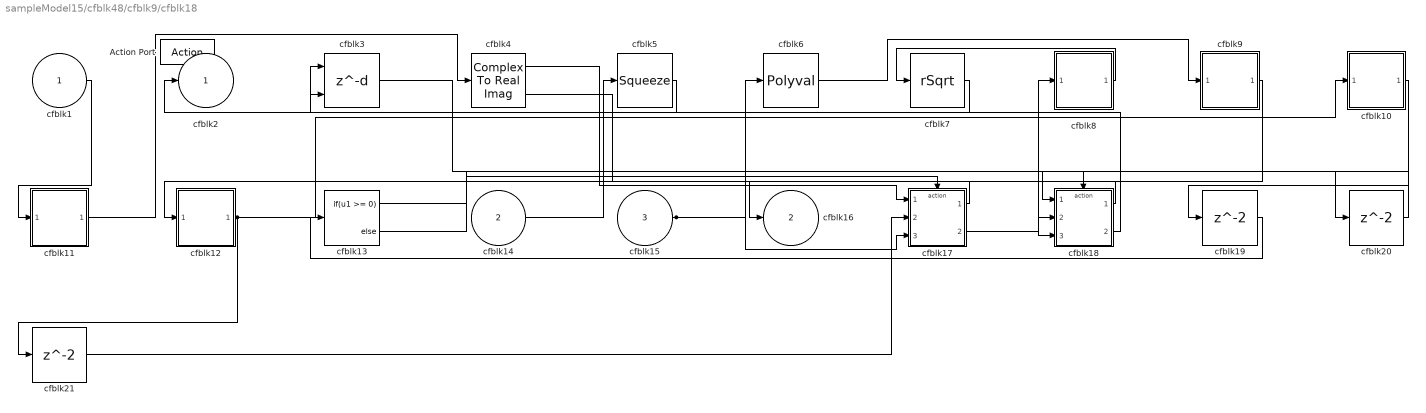
== system sampleModel15/cfblk48/cfblk9/cfblk18 ==
  cfblk1 : Inport
  cfblk14 : Inport  Port=2
  cfblk15 : Inport  Port=3
  Action Port : ActionPort  ActionType=else
  cfblk10 : Subsystem
  cfblk11 : Subsystem
  cfblk12 : Subsystem
  cfblk13 : If  IfExpression=u1 >= 0  SampleTime=1
  cfblk17 : Subsystem  TreatAsAtomicUnit=on
  cfblk18 : Subsystem  TreatAsAtomicUnit=on
  cfblk19 : Delay
  cfblk20 : Delay
  cfblk21 : Delay
  cfblk3 : Delay  DelayLengthSource=Input port
      settings: InputPortMap=u0,p1
  cfblk4 : ComplexToRealImag
  cfblk5 : Squeeze
  cfblk6 : Polyval  Coefs=[ +2.081618890e-019, -1.441693666e-014, +4.719686976e-010, -8.536869453e-006, +1.621573104e-001, -8.087801117e+001 ]
  cfblk7 : Sqrt  Operator=rSqrt  AlgorithmType=Newton-Raphson  SaturateOnIntegerOverflow=on
  cfblk8 : Subsystem
  cfblk9 : Subsystem
  cfblk2 : Outport
  cfblk16 : Outport  Port=2
  wires:
  cfblk1/1 -> cfblk11/1(cfblk1)
  cfblk18/1(cfblk2) -> cfblk16/1
  cfblk8/1(cfblk2) -> cfblk7/1
  cfblk5/1 -> cfblk2/1
  cfblk12/1(cfblk2) -> cfblk10/1(cfblk1), cfblk21/1
  cfblk14/1 -> cfblk5/1
  cfblk18/2(cfblk11) -> cfblk3/1
  cfblk7/1 -> cfblk3/2
  cfblk6/1 -> cfblk9/1(cfblk1)
  cfblk4/1 -> cfblk17/1(cfblk1)
  cfblk17/1(cfblk2) -> cfblk12/1(cfblk1)
  cfblk15/1 -> cfblk6/1, cfblk17/3(cfblk14)
  cfblk11/1(cfblk2) -> cfblk4/1
  cfblk9/1(cfblk2) -> cfblk18/2(cfblk9)
  cfblk4/2 -> cfblk18/3(cfblk10)
  cfblk17/2(cfblk15) -> cfblk8/1(cfblk1)
  cfblk13/1 -> cfblk17/Action
  cfblk13/2 -> cfblk18/Action
  cfblk10/1(cfblk2) -> cfblk19/1
  cfblk19/1 -> cfblk13/1
  cfblk3/1 -> cfblk20/1
  cfblk20/1 -> cfblk18/1(cfblk1)
  cfblk21/1 -> cfblk17/2(cfblk13)

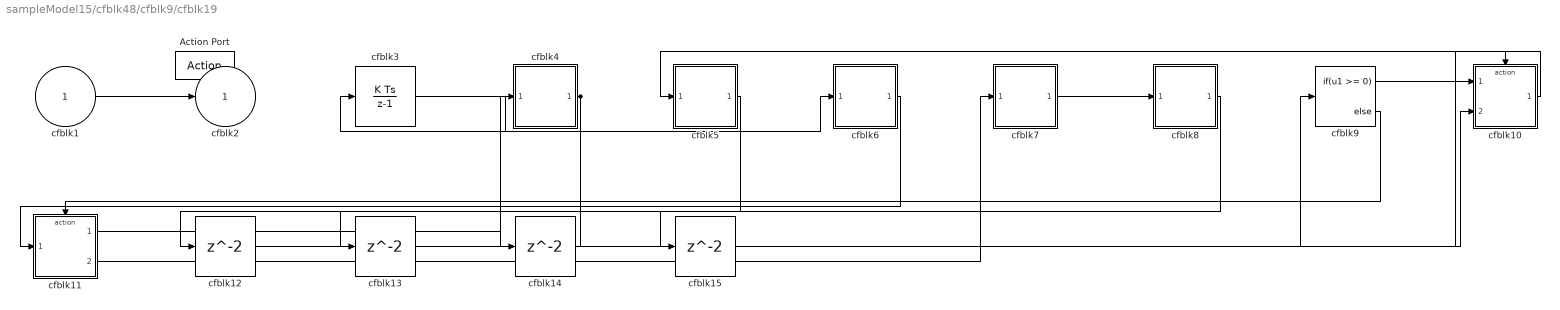
== system sampleModel15/cfblk48/cfblk9/cfblk19 ==
  cfblk1 : Inport
  Action Port : ActionPort  ActionType=then
  cfblk10 : Subsystem  TreatAsAtomicUnit=on
  cfblk11 : Subsystem  TreatAsAtomicUnit=on
  cfblk{12..15} (4 alike) : Delay
  cfblk3 : DiscreteIntegrator  SampleTime=-1  ICPrevOutput=DiscIntNeverNeededParam  ICPrevScaledInput=DiscIntNeverNeededParam
  cfblk4 : Subsystem
  cfblk5 : Subsystem
  cfblk6 : Subsystem
  cfblk7 : Subsystem
  cfblk8 : Subsystem
  cfblk9 : If  IfExpression=u1 >= 0  SampleTime=1
  cfblk2 : Outport
  wires:
  cfblk4/1(cfblk2) -> cfblk13/1, cfblk14/1
  cfblk3/1 -> cfblk6/1(cfblk1)
  cfblk11/1(cfblk2) -> cfblk4/1(cfblk1)
  cfblk1/1 -> cfblk2/1
  cfblk11/2(cfblk15) -> cfblk7/1(cfblk1)
  cfblk10/1(cfblk2) -> cfblk5/1(cfblk1)
  cfblk6/1(cfblk2) -> cfblk11/1(cfblk1)
  cfblk7/1(cfblk2) -> cfblk8/1(cfblk1)
  cfblk9/1 -> cfblk10/Action
  cfblk9/2 -> cfblk11/Action
  cfblk5/1(cfblk2) -> cfblk12/1
  cfblk12/1 -> cfblk10/1(cfblk1)
  cfblk13/1 -> cfblk9/1
  cfblk14/1 -> cfblk3/1
  cfblk8/1(cfblk2) -> cfblk15/1
  cfblk15/1 -> cfblk10/2(cfblk9)

== system sampleModel15/cfblk48/cfblk9/cfblk20 ==
  cfblk1 : Inport
  cfblk11 : Inport  Port=2
  Action Port : ActionPort  ActionType=else
  cfblk10 : Subsystem
  cfblk14 : Delay
  cfblk3 : Trigonometry
  cfblk4 : DotProduct  InputSameDT=on  OutDataTypeStr=Inherit: Inherit via internal rule
  cfblk5 : Assignment  DiagnosticForDimensions=Warning  IndexOptions=Index vector (dialog)  Indices=1  OutputSizes=1
  cfblk6 : Constant  Value=[869315103.100622]  SampleTime=1
  cfblk7 : Subsystem
  cfblk8 : Subsystem
  cfblk9 : Subsystem
  cfblk2 : Outport
  cfblk12 : Outport  Port=2
  cfblk13 : Outport  Port=3
  wires:
  cfblk4/1 -> cfblk5/1
  cfblk3/1 -> cfblk7/1(cfblk1)
  cfblk11/1 -> cfblk13/1
  cfblk1/1 -> cfblk8/1(cfblk1)
  cfblk9/1(cfblk2) -> cfblk12/1
  cfblk10/1(cfblk2) -> cfblk2/1
  cfblk8/1(cfblk2) -> cfblk4/1
  cfblk6/1 -> cfblk4/2, cfblk9/1(cfblk1), cfblk10/1(cfblk1)
  cfblk5/1 -> cfblk3/1
  cfblk7/1(cfblk2) -> cfblk14/1
  cfblk14/1 -> cfblk5/2

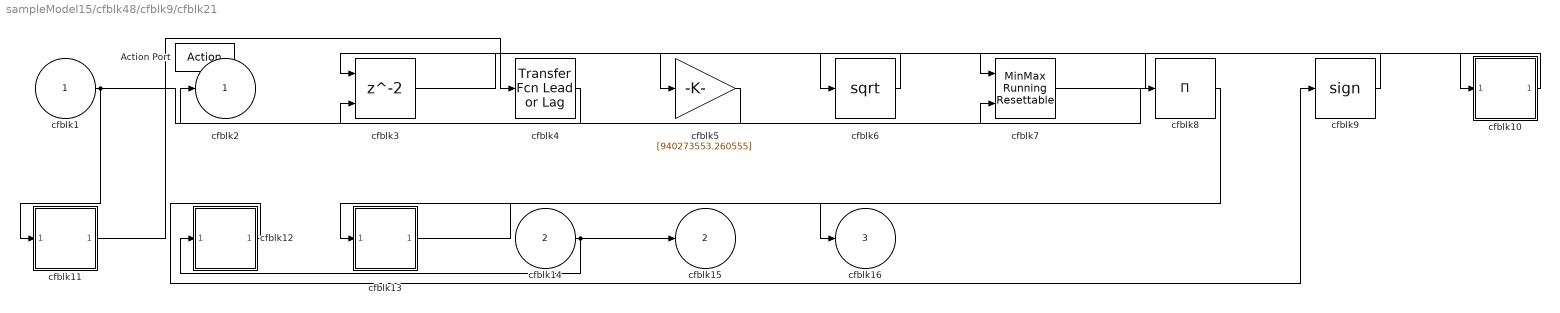
== system sampleModel15/cfblk48/cfblk9/cfblk21 ==
  cfblk1 : Inport
  cfblk14 : Inport  Port=2
  Action Port : ActionPort  ActionType=then
  cfblk10 : Subsystem
  cfblk11 : Subsystem
  cfblk12 : Subsystem
  cfblk13 : Subsystem
  cfblk3 : Delay  ShowEnablePort=on
      settings: InputPortMap=u0,e6
  cfblk4 : simulink/Discrete/Transfer Fcn Lead or Lag  PoleZ=0.95  ZeroZ=0.75  ICPrevOutput=0.0  ICPrevInput=0.0  DoSatur=off
      settings: SourceProductName=Simulink  SourceProductBaseCode=SL
  cfblk5 : Gain  Gain=[940273553.260555]
  cfblk6 : Sqrt  SaturateOnIntegerOverflow=on
  cfblk7 : simulink/Math Operations/MinMax Running Resettable  Function=min  vinit=0.0
  cfblk8 : Product  Inputs=*
  cfblk9 : Signum
  cfblk2 : Outport
  cfblk15 : Outport  Port=2
  cfblk16 : Outport  Port=3
  wires:
  cfblk8/1 -> cfblk13/1(cfblk1)
  cfblk5/1 -> cfblk2/1
  cfblk10/1(cfblk2) -> cfblk5/1
  cfblk9/1 -> cfblk6/1
  cfblk14/1 -> cfblk12/1(cfblk1), cfblk15/1
  cfblk1/1 -> cfblk11/1(cfblk1), cfblk7/2, cfblk8/1
  cfblk13/1(cfblk2) -> cfblk16/1
  cfblk12/1(cfblk2) -> cfblk9/1
  cfblk11/1(cfblk2) -> cfblk4/1
  cfblk6/1 -> cfblk3/1
  cfblk4/1 -> cfblk3/2
  cfblk3/1 -> cfblk7/1
  cfblk7/1 -> cfblk10/1(cfblk1)

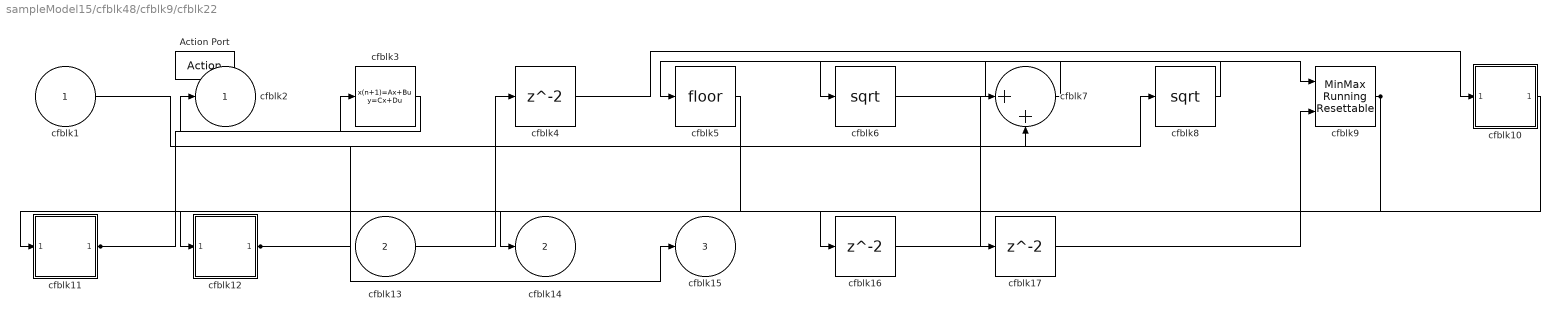
== system sampleModel15/cfblk48/cfblk9/cfblk22 ==
  cfblk1 : Inport
  cfblk13 : Inport  Port=2
  Action Port : ActionPort  ActionType=else
  cfblk10 : Subsystem
  cfblk11 : Subsystem
  cfblk12 : Subsystem
  cfblk16 : Delay
  cfblk17 : Delay
  cfblk3 : DiscreteStateSpace  SampleTime=-1
  cfblk4 : Delay
  cfblk5 : Rounding
  cfblk6 : Sqrt  SaturateOnIntegerOverflow=on
  cfblk7 : Sum  Inputs=|++
  cfblk8 : Sqrt  SaturateOnIntegerOverflow=on
  cfblk9 : simulink/Math Operations/MinMax Running Resettable  Function=min  vinit=0.0
  cfblk2 : Outport
  cfblk14 : Outport  Port=2
  cfblk15 : Outport  Port=3
  wires:
  cfblk10/1(cfblk2) -> cfblk14/1
  cfblk6/1 -> cfblk9/1
  cfblk12/1(cfblk2) -> cfblk15/1, cfblk8/1
  cfblk3/1 -> cfblk2/1
  cfblk9/1 -> cfblk11/1(cfblk1), cfblk16/1
  cfblk7/1 -> cfblk5/1
  cfblk1/1 -> cfblk7/2
  cfblk5/1 -> cfblk12/1(cfblk1)
  cfblk4/1 -> cfblk10/1(cfblk1)
  cfblk8/1 -> cfblk6/1
  cfblk13/1 -> cfblk4/1
  cfblk11/1(cfblk2) -> cfblk3/1, cfblk17/1
  cfblk16/1 -> cfblk7/1
  cfblk17/1 -> cfblk9/2

== system sampleModel15/cfblk48/cfblk9/cfblk6 ==
  cfblk1 : Inport
  cfblk2 : Outport
  wires:
  cfblk1/1 -> cfblk2/1

== system sampleModel15/cfblk48/cfblk9/cfblk7 ==
  cfblk1 : Inport
  cfblk2 : Outport
  wires:
  cfblk1/1 -> cfblk2/1

== system sampleModel15/cfblk48/cfblk9/cfblk8 ==
  cfblk1 : Inport
  cfblk2 : Outport
  wires:
  cfblk1/1 -> cfblk2/1

== system sampleModel15/cfblk48/cfblk9/cfblk17/cfblk11 ==
  cfblk1 : Inport
  cfblk2 : Outport
  wires:
  cfblk1/1 -> cfblk2/1

== system sampleModel15/cfblk48/cfblk9/cfblk17/cfblk12 ==
  cfblk1 : Inport
  cfblk2 : Outport
  wires:
  cfblk1/1 -> cfblk2/1

== system sampleModel15/cfblk48/cfblk9/cfblk17/cfblk13 ==
  cfblk1 : Inport
  cfblk2 : Outport
  wires:
  cfblk1/1 -> cfblk2/1

== system sampleModel15/cfblk48/cfblk9/cfblk18/cfblk10 ==
  cfblk1 : Inport
  cfblk2 : Outport
  wires:
  cfblk1/1 -> cfblk2/1

== system sampleModel15/cfblk48/cfblk9/cfblk18/cfblk11 ==
  cfblk1 : Inport
  cfblk2 : Outport
  wires:
  cfblk1/1 -> cfblk2/1

== system sampleModel15/cfblk48/cfblk9/cfblk18/cfblk12 ==
  cfblk1 : Inport
  cfblk2 : Outport
  wires:
  cfblk1/1 -> cfblk2/1

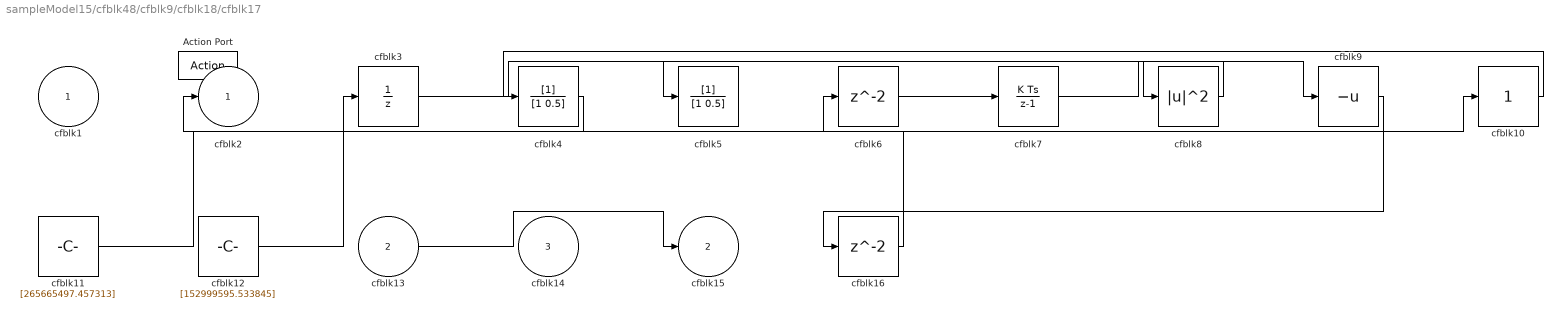
== system sampleModel15/cfblk48/cfblk9/cfblk18/cfblk17 ==
  cfblk1 : Inport
  cfblk13 : Inport  Port=2
  cfblk14 : Inport  Port=3
  Action Port : ActionPort  ActionType=then
  cfblk10 : simulink/Math Operations/Slider Gain  gain=1  low=0  high=2
  cfblk11 : Constant  Value=[265665497.457313]  SampleTime=1
  cfblk12 : Constant  Value=[152999595.533845]  SampleTime=1
  cfblk16 : Delay
  cfblk3 : UnitDelay  SampleTime=-1
  cfblk4 : DiscreteFilter
  cfblk5 : DiscreteFilter
  cfblk6 : Delay
  cfblk7 : DiscreteIntegrator  SampleTime=-1  ICPrevOutput=DiscIntNeverNeededParam  ICPrevScaledInput=DiscIntNeverNeededParam
  cfblk8 : Math  Operator=magnitude^2  SaturateOnIntegerOverflow=on
  cfblk9 : UnaryMinus
  cfblk2 : Outport
  cfblk15 : Outport  Port=2
  wires:
  cfblk3/1 -> cfblk8/1
  cfblk11/1 -> cfblk10/1
  cfblk4/1 -> cfblk2/1
  cfblk8/1 -> cfblk5/1
  cfblk6/1 -> cfblk7/1
  cfblk13/1 -> cfblk15/1
  cfblk10/1 -> cfblk4/1
  cfblk12/1 -> cfblk3/1
  cfblk7/1 -> cfblk9/1
  cfblk9/1 -> cfblk16/1
  cfblk16/1 -> cfblk6/1

== system sampleModel15/cfblk48/cfblk9/cfblk18/cfblk18 ==
  cfblk1 : Inport
  cfblk9 : Inport  Port=2
  cfblk10 : Inport  Port=3
  Action Port : ActionPort  ActionType=else
  cfblk12 : Delay
  cfblk3 : simulink/Continuous/PID Controller (2DOF)  Controller=PID  TimeDomain=Discrete-time  SampleTime=-1  IntegratorMethod=Forward Euler  FilterMethod=Forward Euler  Form=Parallel  UseFilter=on  ControllerParametersSource=internal  P=1  I=1  D=0  N=100  b=1  c=1  InitialConditionSource=internal  InitialConditionForIntegrator=0  InitialConditionForFilter=0  ExternalReset=none  LimitOutput=off  UpperSaturationLimit=inf  LowerSaturationLimit=-inf  LinearizeAsGain=off  AntiWindupMode=none  Kb=1  TrackingMode=off  Kt=1  PParamMin=[]  PParamMax=[]  IParamMin=[]  IParamMax=[]  DParamMin=[]  DParamMax=[]  NParamMin=[]  NParamMax=[]  bParamMin=[]  bParamMax=[]  cParamMin=[]  cParamMax=[]  KbParamMin=[]  KbParamMax=[]  KtParamMin=[]  KtParamMax=[]  POutMin=[]  POutMax=[]  IOutMin=[]  IOutMax=[]  DOutMin=[]  DOutMax=[]  NOutMin=[]  NOutMax=[]  bOutMin=[]  bOutMax=[]  cOutMin=[]  cOutMax=[]  KbOutMin=[]  KbOutMax=[]  KtOutMin=[]  KtOutMax=[]  IntegratorOutMin=[]  IntegratorOutMax=[]  FilterOutMin=[]  FilterOutMax=[]  SumOutMin=[]  SumOutMax=[]  Sum1OutMin=[]  Sum1OutMax=[]  Sum2OutMin=[]  Sum2OutMax=[]  Sum3OutMin=[]  Sum3OutMax=[]  SumI1OutMin=[]  SumI1OutMax=[]  SumI2OutMin=[]  SumI2OutMax=[]  SumI3OutMin=[]  SumI3OutMax=[]  SumDOutMin=[]  SumDOutMax=[]  SaturationOutMin=[]  SaturationOutMax=[]  IntegratorContinuousStateAttributes=''  IntegratorStateMustResolveToSignalObject=off  IntegratorRTWStateStorageClass=Auto  FilterContinuousStateAttributes=''  FilterStateMustResolveToSignalObject=off  FilterRTWStateStorageClass=Auto  DifferentiatorICPrevScaledInput=0  DifferentiatorOutMin=[]  DifferentiatorOutMax=[]  FilterDiffOutCoefMin=[]  FilterDiffOutCoefMax=[]  SumDenOutMin=[]  SumDenOutMax=[]  SumNumOutMin=[]  SumNumOutMax=[]  ReciprocalOutMin=[]  ReciprocalOutMax=[]  DivideOutMin=[]  DivideOutMax=[]  TunerSelectOption=Transfer Function Based (PID Tuner App)
  cfblk4 : simulink/Discrete/Transfer Fcn Lead or Lag  PoleZ=0.95  ZeroZ=0.75  ICPrevOutput=0.0  ICPrevInput=0.0  DoSatur=off
      settings: SourceProductName=Simulink  SourceProductBaseCode=SL
  cfblk5 : DiscreteStateSpace  SampleTime=-1
  cfblk6 : Trigonometry
  cfblk7 : Sqrt  Operator=rSqrt  AlgorithmType=Newton-Raphson  SaturateOnIntegerOverflow=on
  cfblk8 : Assignment  DiagnosticForDimensions=Warning  IndexOptions=Index vector (dialog)  Indices=1  OutputSizes=1
  cfblk2 : Outport
  cfblk11 : Outport  Port=2
  wires:
  cfblk1/1 -> cfblk11/1
  cfblk5/1 -> cfblk4/1
  cfblk7/1 -> cfblk3/1
  cfblk6/1 -> cfblk8/1
  cfblk4/1 -> cfblk7/1
  cfblk10/1 -> cfblk5/1
  cfblk3/1 -> cfblk2/1
  cfblk9/1 -> cfblk8/2
  cfblk8/1 -> cfblk3/2, cfblk12/1
  cfblk12/1 -> cfblk6/1

== system sampleModel15/cfblk48/cfblk9/cfblk18/cfblk8 ==
  cfblk1 : Inport
  cfblk2 : Outport
  wires:
  cfblk1/1 -> cfblk2/1

== system sampleModel15/cfblk48/cfblk9/cfblk18/cfblk9 ==
  cfblk1 : Inport
  cfblk2 : Outport
  wires:
  cfblk1/1 -> cfblk2/1

== system sampleModel15/cfblk48/cfblk9/cfblk19/cfblk10 ==
  cfblk1 : Inport
  cfblk9 : Inport  Port=2
  Action Port : ActionPort  ActionType=then
  cfblk10 : Delay
  cfblk3 : UnitDelay  SampleTime=-1
  cfblk4 : Product
  cfblk5 : Signum
  cfblk6 : DotProduct  InputSameDT=on  OutDataTypeStr=Inherit: Inherit via internal rule
  cfblk7 : UnaryMinus
  cfblk8 : Constant  Value=[415745499.794823]  SampleTime=1
  cfblk2 : Outport
  wires:
  cfblk7/1 -> cfblk6/1
  cfblk9/1 -> cfblk5/1
  cfblk8/1 -> cfblk4/1
  cfblk5/1 -> cfblk6/2
  cfblk3/1 -> cfblk4/2
  cfblk6/1 -> cfblk2/1
  cfblk1/1 -> cfblk7/1
  cfblk4/1 -> cfblk10/1
  cfblk10/1 -> cfblk3/1

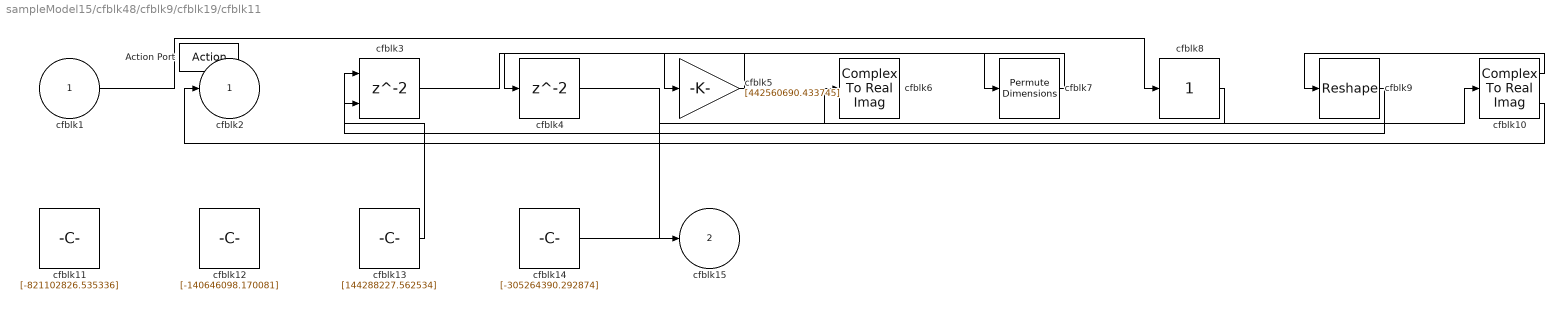
== system sampleModel15/cfblk48/cfblk9/cfblk19/cfblk11 ==
  cfblk1 : Inport
  Action Port : ActionPort  ActionType=else
  cfblk10 : ComplexToRealImag
  cfblk11 : Constant  Value=[-821102826.535336]  SampleTime=1
  cfblk12 : Constant  Value=[-140646098.170081]  SampleTime=1
  cfblk13 : Constant  Value=[144288227.562534]  SampleTime=1
  cfblk14 : Constant  Value=[-305264390.292874]  SampleTime=1
  cfblk3 : Delay  ShowEnablePort=on
      settings: InputPortMap=u0,e6
  cfblk4 : Delay
  cfblk5 : Gain  Gain=[442560690.433745]
  cfblk6 : ComplexToRealImag
  cfblk7 : PermuteDimensions
  cfblk8 : simulink/Math Operations/Slider Gain  gain=1  low=0  high=2
  cfblk9 : Reshape
  cfblk2 : Outport
  cfblk15 : Outport  Port=2
  wires:
  cfblk10/1 -> cfblk9/1
  cfblk7/1 -> cfblk5/1
  cfblk8/1 -> cfblk6/1
  cfblk9/1 -> cfblk3/1
  cfblk10/2 -> cfblk2/1
  cfblk13/1 -> cfblk3/2
  cfblk4/1 -> cfblk15/1
  cfblk14/1 -> cfblk10/1
  cfblk1/1 -> cfblk8/1
  cfblk5/1 -> cfblk4/1
  cfblk3/1 -> cfblk7/1

== system sampleModel15/cfblk48/cfblk9/cfblk19/cfblk4 ==
  cfblk1 : Inport
  cfblk2 : Outport
  wires:
  cfblk1/1 -> cfblk2/1

== system sampleModel15/cfblk48/cfblk9/cfblk19/cfblk5 ==
  cfblk1 : Inport
  cfblk2 : Outport
  wires:
  cfblk1/1 -> cfblk2/1

== system sampleModel15/cfblk48/cfblk9/cfblk19/cfblk6 ==
  cfblk1 : Inport
  cfblk2 : Outport
  wires:
  cfblk1/1 -> cfblk2/1

== system sampleModel15/cfblk48/cfblk9/cfblk19/cfblk7 ==
  cfblk1 : Inport
  cfblk2 : Outport
  wires:
  cfblk1/1 -> cfblk2/1

== system sampleModel15/cfblk48/cfblk9/cfblk19/cfblk8 ==
  cfblk1 : Inport
  cfblk2 : Outport
  wires:
  cfblk1/1 -> cfblk2/1

== system sampleModel15/cfblk48/cfblk9/cfblk20/cfblk10 ==
  cfblk1 : Inport
  cfblk2 : Outport
  wires:
  cfblk1/1 -> cfblk2/1

== system sampleModel15/cfblk48/cfblk9/cfblk20/cfblk7 ==
  cfblk1 : Inport
  cfblk2 : Outport
  wires:
  cfblk1/1 -> cfblk2/1

== system sampleModel15/cfblk48/cfblk9/cfblk20/cfblk8 ==
  cfblk1 : Inport
  cfblk2 : Outport
  wires:
  cfblk1/1 -> cfblk2/1

== system sampleModel15/cfblk48/cfblk9/cfblk20/cfblk9 ==
  cfblk1 : Inport
  cfblk2 : Outport
  wires:
  cfblk1/1 -> cfblk2/1

== system sampleModel15/cfblk48/cfblk9/cfblk21/cfblk10 ==
  cfblk1 : Inport
  cfblk2 : Outport
  wires:
  cfblk1/1 -> cfblk2/1

== system sampleModel15/cfblk48/cfblk9/cfblk21/cfblk11 ==
  cfblk1 : Inport
  cfblk2 : Outport
  wires:
  cfblk1/1 -> cfblk2/1

== system sampleModel15/cfblk48/cfblk9/cfblk21/cfblk12 ==
  cfblk1 : Inport
  cfblk2 : Outport
  wires:
  cfblk1/1 -> cfblk2/1

== system sampleModel15/cfblk48/cfblk9/cfblk21/cfblk13 ==
  cfblk1 : Inport
  cfblk2 : Outport
  wires:
  cfblk1/1 -> cfblk2/1

== system sampleModel15/cfblk48/cfblk9/cfblk22/cfblk10 ==
  cfblk1 : Inport
  cfblk2 : Outport
  wires:
  cfblk1/1 -> cfblk2/1

== system sampleModel15/cfblk48/cfblk9/cfblk22/cfblk11 ==
  cfblk1 : Inport
  cfblk2 : Outport
  wires:
  cfblk1/1 -> cfblk2/1

== system sampleModel15/cfblk48/cfblk9/cfblk22/cfblk12 ==
  cfblk1 : Inport
  cfblk2 : Outport
  wires:
  cfblk1/1 -> cfblk2/1
